simulink library "Library_RCelements"  (Simulink 4.00)
settings Model: Creator=Felipe Aristizabal  LastModifiedBy=felipe

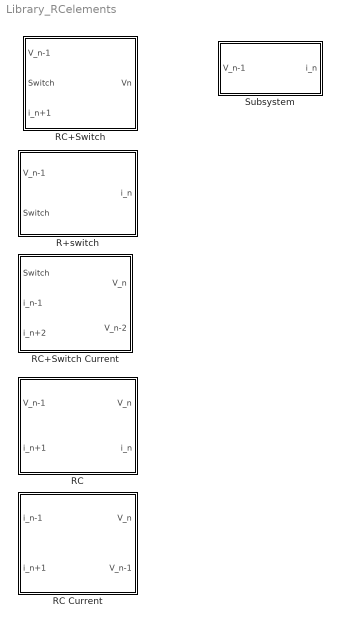
== system Library_RCelements ==
  R+switch : Subsystem  mask(Switch plus Resistor){R1=}
      mask prompts: R1 "Resistance R"
      mask init:
      | x1 = [0.1 0.2 0.21:.02:0.43 0.44 0.6]+0.1;
      | y1= [0.8 0.8 0.85 0.75 0.85 0.75 0.85 0.75 0.85 0.75 0.85 0.75 0.85 0.75 0.80 0.80];
      | x2 = [0.2 0.7];
      | y2 = [0.2 0.2];
      | x3 = [0.7 0.7];
      | x4 = [0.7 0.7];
      | y3 = [0.8 0.6];
      | y4 = [0.45 0.2];
      | x5 = [0.7 0.77];
      | y5 = [0.6 0.4];
      settings: RTWFcnNameOpts=Auto  RTWFileNameOpts=Auto
      mask Display:
      | plot(x1,y1, x2, y2);
      | plot(x3,y3);
      | plot(x4,y4);
      | plot(x5,y5);
  RC : Subsystem  mask(Single RC){Rn=, Cn=, initVal=}
      mask prompts: Rn "Resistance"; Cn "Capacitance"; initVal "Initial Voltage accross the condensor"
      mask help: Single RC element
      mask init:
      | x1 = [0.1 0.2 0.21:.02:0.43 0.44 0.7]+0.1;
      | y1= [0.8 0.8 0.85 0.75 0.85 0.75 0.85 0.75 0.85 0.75 0.85 0.75 0.85 0.75 0.80 0.80];
      | x2 = [0.2 0.8];
      | y2 = [0.2 0.2];
      | x3 = [0.7 0.7];
      | x4 = [0.7 0.7];
      | y3 = [0.8 0.6];
      | y4 = [0.55 0.2];
      | x5 = [0.63 0.77];
      | y5 = [0.6 0.6];
      | x6 = [0.63 0.77];
      | y6 = [0.55 0.55];
      settings: RTWFcnNameOpts=Auto  RTWFileNameOpts=Auto
      mask Display:
      | plot(x1,y1, x2, y2);
      | plot(x3,y3);
      | plot(x4,y4);
      | plot(x5,y5);
      | plot(x6,y6);
  RC Current : Subsystem  AncestorBlock=Library_RCelements/RC  mask(Single RC){Rn=10, Cn=0.02, initVal=0}
      mask prompts: Rn "Resistance"; Cn "Capacitance"; initVal "Initial Voltage accross the condensor"
      mask help: Single RC element
      mask init:
      | x1 = [0.1 0.2 0.21:.02:0.43 0.44 0.7]+0.1;
      | y1= [0.8 0.8 0.85 0.75 0.85 0.75 0.85 0.75 0.85 0.75 0.85 0.75 0.85 0.75 0.80 0.80];
      | x2 = [0.2 0.8];
      | y2 = [0.2 0.2];
      | x3 = [0.7 0.7];
      | x4 = [0.7 0.7];
      | y3 = [0.8 0.6];
      | y4 = [0.55 0.2];
      | x5 = [0.63 0.77];
      | y5 = [0.6 0.6];
      | x6 = [0.63 0.77];
      | y6 = [0.55 0.55];
      | t = [0:0.1:2*pi, 2*pi];
      | x = 0.1*cos(t) + 0.3;
      | y = 0.1*sin(t) + 0.5;
      | x7 = [0.27 0.33 NaN 0.27 0.33 NaN 0.3 0.3];
      | y7 = [0.45 0.45 NaN 0.55 0.55 NaN 0.45 0.55];
      settings: RTWFcnNameOpts=Auto  RTWFileNameOpts=Auto
      mask Display:
      | plot(x1,y1, x2, y2);
      | plot(x3,y3);
      | plot(x4,y4);
      | plot(x5,y5);
      | plot(x6,y6);
      | plot(x,y);
      | plot(x7,y7)
  RC+Switch : Subsystem  mask(RC + Switch){R=, C=, V0=}
      mask prompts: R "Resisatnce"; C "Capacitance"; V0 "Initial Voltage"
      mask init:
      | x1= [0.1 0.2 0.21 0.23 0.25 0.27 0.29 0.31 0.33 0.34 0.40 0.50]+0.1;
      | y1= [0.8 0.8 0.85 0.75 0.85 0.75 0.85 0.75 0.85 0.80 0.80 0.90];
      | x11 = [0.60 0.8];
      | y11 = [0.8 0.8];
      | x2 = [0.2 0.8];
      | y2 = [0.2 0.2];
      | x3 = [0.7 0.7];
      | x4 = [0.7 0.7];
      | y3 = [0.8 0.6];
      | y4 = [0.55 0.2];
      | x5 = [0.63 0.77];
      | y5 = [0.6 0.6];
      | x6 = [0.63 0.77];
      | y6 = [0.55 0.55];
      settings: RTWFcnNameOpts=Auto  RTWFileNameOpts=Auto
      mask Display:
      | plot(x1,y1, x2, y2, x11, y11);
      | plot(x3,y3);
      | plot(x4,y4);
      | plot(x5,y5);
      | plot(x6,y6);
  RC+Switch Current : Subsystem  AncestorBlock=Library_RCelements/RC+Switch  mask(RC + Switch){Rn=10, Cn=0.2, V0=0}
      mask prompts: Rn "Resisatnce"; Cn "Capacitance"; V0 "Initial Voltage"
      mask init:
      | x1= [0.1 0.2 0.21 0.23 0.25 0.27 0.29 0.31 0.33 0.34 0.40 0.50]+0.1;
      | y1= [0.8 0.8 0.85 0.75 0.85 0.75 0.85 0.75 0.85 0.80 0.80 0.90];
      | x11 = [0.60 0.8];
      | y11 = [0.8 0.8];
      | x2 = [0.2 0.8];
      | y2 = [0.2 0.2];
      | x3 = [0.7 0.7];
      | x4 = [0.7 0.7];
      | y3 = [0.8 0.6];
      | y4 = [0.55 0.2];
      | x5 = [0.63 0.77];
      | y5 = [0.6 0.6];
      | x6 = [0.63 0.77];
      | y6 = [0.55 0.55];
      | t = [0:0.1:2*pi, 2*pi];
      | x = 0.1*cos(t) + 0.3;
      | y = 0.1*sin(t) + 0.5;
      | x7 = [0.27 0.33 NaN 0.27 0.33 NaN 0.3 0.3];
      | y7 = [0.45 0.45 NaN 0.55 0.55 NaN 0.45 0.55];
      settings: RTWFcnNameOpts=Auto  RTWFileNameOpts=Auto
      mask Display:
      | plot(x1,y1, x2, y2, x11, y11);
      | plot(x3,y3);
      | plot(x4,y4);
      | plot(x5,y5);
      | plot(x6,y6);
      | plot(x,y);
      | plot(x7,y7)
  Subsystem : Subsystem  mask{V2=, R1=}
      mask prompts: V2 "Source Voltage"; R1 "Resistance R1"
      mask init:
      | x1 = [0.1 0.2 0.21:.02:0.43 0.44 0.6]+0.1;
      | y1= [0.8 0.8 0.85 0.75 0.85 0.75 0.85 0.75 0.85 0.75 0.85 0.75 0.85 0.75 0.80 0.80];
      | x2 = [0.2 0.7];
      | y2 = [0.2 0.2];
      | x3 = [0.7 0.7];
      | x4 = [0.7 0.7];
      | y3 = [0.8 0.6];
      | y4 = [0.50 0.2];
      | x5 = [0.63 0.77];
      | y5 = [0.6 0.6];
      | x6 = [0.58 0.82];
      | y6 = [0.50 0.50];
      settings: RTWFcnNameOpts=Auto  RTWFileNameOpts=Auto
      mask Display:
      | plot(x1,y1, x2, y2);
      | plot(x3,y3);
      | plot(x4,y4);
      | plot(x5,y5);
      | plot(x6,y6);

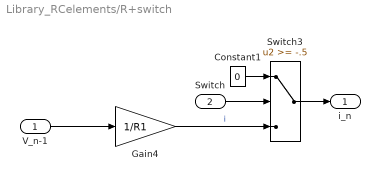
== system Library_RCelements/R+switch ==
  V_n-1 : Inport  Port=1
  Switch : Inport  Port=2
  Constant1 : Constant  Value=0
  Gain4 : Gain  Gain=1/R1  Multiplication=Element-wise(K.*u)  SaturateOnIntegerOverflow=on
  Switch3 : Switch  Threshold=-.5
  i_n : Outport  Port=1
  wires:
  V_n-1/1 -> Gain4/1
  Switch3/1 -> i_n/1
  Gain4/1 -> Switch3/3  "i"
  Switch/1 -> Switch3/2
  Constant1/1 -> Switch3/1

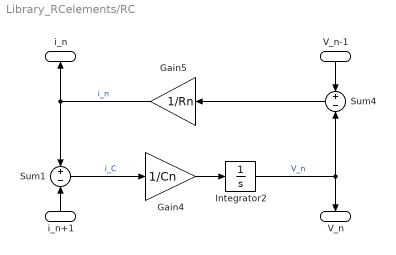
== system Library_RCelements/RC ==
  V_n-1 : Inport  Orientation=down  Port=1
  i_n+1 : Inport  Orientation=up  Port=2
  Gain4 : Gain  Gain=1/Cn  Multiplication=Element-wise(K.*u)  SaturateOnIntegerOverflow=on
  Gain5 : Gain  Orientation=left  Gain=1/Rn  Multiplication=Element-wise(K.*u)  SaturateOnIntegerOverflow=on
  Integrator2 : Integrator  ExternalReset=none  InitialConditionSource=internal  InitialCondition=initVal  LimitOutput=off  UpperSaturationLimit=inf  LowerSaturationLimit=-inf  ShowSaturationPort=off  ShowStatePort=off  AbsoluteTolerance=auto
  Sum1 : Sum  Inputs=+-  SaturateOnIntegerOverflow=on
  Sum4 : Sum  Orientation=left  Inputs=+-  SaturateOnIntegerOverflow=on
  V_n : Outport  Orientation=down  Port=1
  i_n : Outport  Orientation=up  Port=2
  wires:
  i_n+1/1 -> Sum1/2
  Gain5/1 -> i_n/1, Sum1/1  "i_n"
  Sum1/1 -> Gain4/1  "i_C"
  Integrator2/1 -> V_n/1, Sum4/2  "V_n"
  V_n-1/1 -> Sum4/1
  Gain4/1 -> Integrator2/1
  Sum4/1 -> Gain5/1

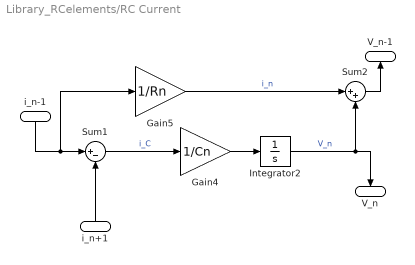
== system Library_RCelements/RC Current ==
  i_n-1 : Inport  Orientation=down  Port=1
  i_n+1 : Inport  Orientation=up  Port=2
  Gain4 : Gain  Gain=1/Cn  Multiplication=Element-wise(K.*u)  SaturateOnIntegerOverflow=on
  Gain5 : Gain  Gain=1/Rn  Multiplication=Element-wise(K.*u)  SaturateOnIntegerOverflow=on
  Integrator2 : Integrator  ExternalReset=none  InitialConditionSource=internal  InitialCondition=initVal  LimitOutput=off  UpperSaturationLimit=inf  LowerSaturationLimit=-inf  ShowSaturationPort=off  ShowStatePort=off  AbsoluteTolerance=auto
  Sum1 : Sum  Inputs=|+-  SaturateOnIntegerOverflow=on
  Sum2 : Sum  Inputs=|++  SaturateOnIntegerOverflow=on
  V_n : Outport  Orientation=down  Port=1
  V_n-1 : Outport  Orientation=up  Port=2
  wires:
  Sum2/1 -> V_n-1/1
  Gain5/1 -> Sum2/1  "i_n"
  i_n-1/1 -> Gain5/1, Sum1/1
  i_n+1/1 -> Sum1/2
  Sum1/1 -> Gain4/1  "i_C"
  Integrator2/1 -> Sum2/2, V_n/1  "V_n"
  Gain4/1 -> Integrator2/1

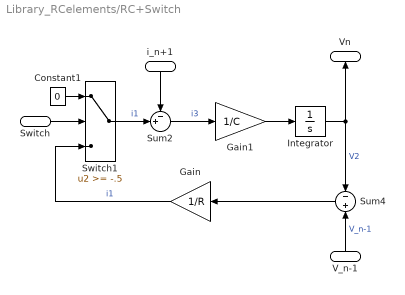
== system Library_RCelements/RC+Switch ==
  V_n-1 : Inport  Orientation=up  Port=1
  Switch : Inport  Port=2
  i_n+1 : Inport  Orientation=down  Port=3
  Constant1 : Constant  Value=0
  Gain : Gain  Orientation=left  Gain=1/R  Multiplication=Element-wise(K.*u)  SaturateOnIntegerOverflow=on
  Gain1 : Gain  Gain=1/C  Multiplication=Element-wise(K.*u)  SaturateOnIntegerOverflow=on
  Integrator : Integrator  ExternalReset=none  InitialConditionSource=internal  InitialCondition=V0  LimitOutput=off  UpperSaturationLimit=inf  LowerSaturationLimit=-inf  ShowSaturationPort=off  ShowStatePort=off  AbsoluteTolerance=auto
  Sum2 : Sum  Inputs=-+|  SaturateOnIntegerOverflow=on
  Sum4 : Sum  Orientation=left  Inputs=-+  SaturateOnIntegerOverflow=on
  Switch1 : Switch  Threshold=-.5
  Vn : Outport  Orientation=up  Port=1
  wires:
  i_n+1/1 -> Sum2/1
  Sum4/1 -> Gain/1
  V_n-1/1 -> Sum4/2  "V_n-1"
  Switch1/1 -> Sum2/2  "i1"
  Gain/1 -> Switch1/3  "i1"
  Constant1/1 -> Switch1/1
  Sum2/1 -> Gain1/1  "i3"
  Integrator/1 -> Vn/1, Sum4/1  "V2"
  Gain1/1 -> Integrator/1
  Switch/1 -> Switch1/2

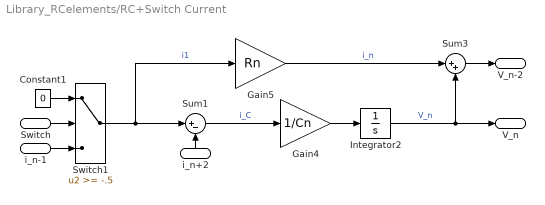
== system Library_RCelements/RC+Switch Current ==
  Switch : Inport  Port=1
  i_n-1 : Inport  Port=2
  i_n+2 : Inport  Orientation=up  Port=3
  Constant1 : Constant  Value=0
  Gain4 : Gain  Gain=1/Cn  Multiplication=Element-wise(K.*u)  SaturateOnIntegerOverflow=on
  Gain5 : Gain  Gain=Rn  Multiplication=Element-wise(K.*u)  SaturateOnIntegerOverflow=on
  Integrator2 : Integrator  ExternalReset=none  InitialConditionSource=internal  InitialCondition=V0  LimitOutput=off  UpperSaturationLimit=inf  LowerSaturationLimit=-inf  ShowSaturationPort=off  ShowStatePort=off  AbsoluteTolerance=auto
  Sum1 : Sum  Inputs=|+-  SaturateOnIntegerOverflow=on
  Sum3 : Sum  Inputs=|++  SaturateOnIntegerOverflow=on
  Switch1 : Switch  Threshold=-.5
  V_n : Outport  Port=1
  V_n-2 : Outport  Port=2
  wires:
  i_n-1/1 -> Switch1/3
  Switch1/1 -> Gain5/1, Sum1/1  "i1"
  Gain4/1 -> Integrator2/1
  Integrator2/1 -> Sum3/2, V_n/1  "V_n"
  Sum1/1 -> Gain4/1  "i_C"
  i_n+2/1 -> Sum1/2
  Gain5/1 -> Sum3/1  "i_n"
  Sum3/1 -> V_n-2/1
  Constant1/1 -> Switch1/1
  Switch/1 -> Switch1/2

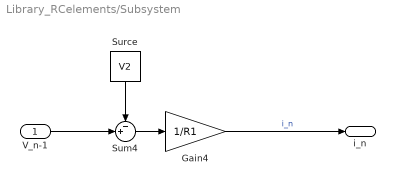
== system Library_RCelements/Subsystem ==
  V_n-1 : Inport  Port=1
  Gain4 : Gain  Gain=1/R1  Multiplication=Element-wise(K.*u)  SaturateOnIntegerOverflow=on
  Sum4 : Sum  Inputs=-+|  SaturateOnIntegerOverflow=on
  Surce : Constant  Orientation=down  Value=V2
  i_n : Outport  Port=1
  wires:
  Gain4/1 -> i_n/1  "i_n"
  Sum4/1 -> Gain4/1
  Surce/1 -> Sum4/1
  V_n-1/1 -> Sum4/2
